simulink model "proyecto_c_fc1"  (R2023b)
settings: Solver=VariableStepAuto  StartTime=0.0  StopTime=0.1  RelTol=1e-3
values from neighbouring files (symbols this model uses):
  test_fs = 10*test_FI    (= 1100000)    [simulink_parametros.m]
  test_ts = 1/test_fs    (= 9.09090909091e-07)    [simulink_parametros.m]
undefined symbols (not defined in the file or in its folder): fdesignblkfcn, gcbh, salida_sintonizador_fc1
(part 2 of 3)

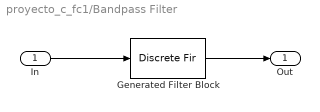
== system proyecto_c_fc1/Bandpass Filter ==
  In : Inport
  Generated Filter Block : DiscreteFir  Tag=BlockMethodSubSystem  Coefficients=[-1.1273741661103097e-05 -0.000561993375017939118 -8.62359604901059074e-06 -7.50691451952865943e-06 7.81285012600206921e-06 2.00315466230824187e-05 2.45542488551999855e-05 1.96579514985156776e-05 7.23640037101240103e-06 -7.77377859031782842e-06 -1.95786442923720696e-05 -2.36211150463387239e-05 -1.85928598378592355e-05 -6.64846825538893349e-06 7.29488094785432066e-06 1.78537303848593843e-05 2.10687862697230246e-05 1.61984502957142459e-05 5.57043766828194584e-06 -6.2241917677792999e-06 -1.46271891284538723e-05 -1.66402961373941308e-05 -1.22566929648169262e-05 -3.87374512389737483e-06 4.58454412376723479e-06 9.84138810207142664e-06 1.02519398320708616e-05 6.71871312055139123e-06 1.58809022200205806e-06 -2.2582235367900078e-06 -3.31668402739260329e-06 -1.71057390280937806e-06 5.71415080786260673e-07 1.37365127836489052e-06 -7.40243038831310612e-07 -4.98291161961237695e-06 -9.03558948382597868e-06 -9.64922274212810738e-06 -5.01330364005861426e-06 4.44329105706563102e-06 1.5111667798730986e-05 2.20480416378027126e-05 2.05718981177941884e-05 9.37944450890057011e-06 -8.81327587071295006e-06 -2.7044796185290007e-05 -3.73199178557717198e-05 -3.33531572241261174e-05 -1.45052551295041108e-05 1.38085893311933062e-05 4.07441787704725277e-05 5.48266852961340758e-05 4.79728578235877378e-05 2.03548411190195869e-05 -1.95098536092251836e-05 -5.63373604246019405e-05 -7.47121602266063008e-05 -6.45057530590528396e-05 -2.6848117468770755e-05 2.62185647654078497e-05 7.42846473933374068e-05 9.74383073049243437e-05 8.31269841312136181e-05 3.38624577328217678e-05 -3.37557972285601769e-05 -9.28593154031518651e-05 -0.000121715883273213274 -0.000103110631245326945 -4.18434112008373021e-05 4.11800005301413355e-05 0.000114539986861578346 0.000147886559587942322 0.000124842081019382889 5.0328045572193971e-05 -4.96937409930004861e-05 -0.000137103551268169966 -0.000176221348144385667 -0.000148056062433894135 -5.93670418374609682e-05 5.8693902067989684e-05 0.000161023583209106517 0.00020615499807303598 0.000172524825800646577 6.88269154916930148e-05 -6.82044774625502093e-05 -0.000186161062629007431 -0.000237511838074231984 -0.000198103723660641512 -7.87069884315816072e-05 7.80569319854972261e-05 0.00021219548486503786 0.000269918913074930456 0.000224479149824362284 8.88582642268017563e-05 -8.81992874037328524e-05 -0.000238908101307476863 -0.00030309523201981647 -0.000251435206871207116 -9.92380030659086661e-05 9.84601613227532272e-05 0.000265950476991421011 0.000336621971429807202 0.000278615840106215566 0.000109667442667640356 -0.000108789263597097103 -0.00029307244102745898 -0.000370151804034989562 -0.00030571705306141106 -0.00012001470511117765 0.000119078850272852995 0.000319949942657759667 0.000403257314825242663 0.000332373280653635867 0.000130128999717177149 -0.000129191397318941626 -0.000346207439079053349 -0.000435487167876184172 -0.000358270010401962003 -0.000139995158263942821 0.000138808262929293846 0.00037130910355592274 0.000466285513354377167 0.000383001680404604025 0.000149397396889170054 -0.000148013856622131011 -0.000395256594413965665 -0.000495470830329233997 -0.000406154867513150496 -0.000158003610846158552 0.000156489143938728231 0.000417360887721305782 0.000522275276674819228 0.00042747622293450694 0.000166119588584539072 -0.000164461364275621599 -0.000437267726654737602 -0.000546432609467402018 -0.000446541285845892752 -0.00017317798670501736 0.000171370443118935731 0.000454848435996221974 0.000567483644046186094 0.000463034717222465201 0.000179262482419011903 -0.000177234027989062962 -0.000469626690795197689 -0.000585015187900282826 -0.000476610184146802874 -0.000184202970080055817 0.000181966563408566666 0.000481351002765526394 0.000598701097780842111 0.000487018917664339406 0.000187921767392541512 -0.000185431904334681312 -0.000489721519980618062 -0.000608177780856590001 -0.000493960052418473852 -0.000190273004724368763 0.00018758784085693404 0.000494550609676252043 0.00061320692442606232 0.000497254875120825448 0.000191215063734824497 ...(+101361 chars)]  InputProcessing=Columns as channels (frame based)
  Out : Outport  VectorParamsAs1DForOutWhenUnconnected=off
  wires:
  In/1 -> Generated Filter Block/1
  Generated Filter Block/1 -> Out/1
